simulink model "BallPlate_FLControl"  (R2018b)
settings: Solver=FixedStepAuto  StartTime=0.0  StopTime=20  FixedStep=0.01  RelTol=1e-5
undefined symbols (not defined in the file or in its folder): K
libraries: vrlib x42, simulink x5, aerolibanimutils x3, powerlib_meascontrol x1
(part 1 of 2)
settings Model: Creator=enrico  LastModifiedBy=Dan

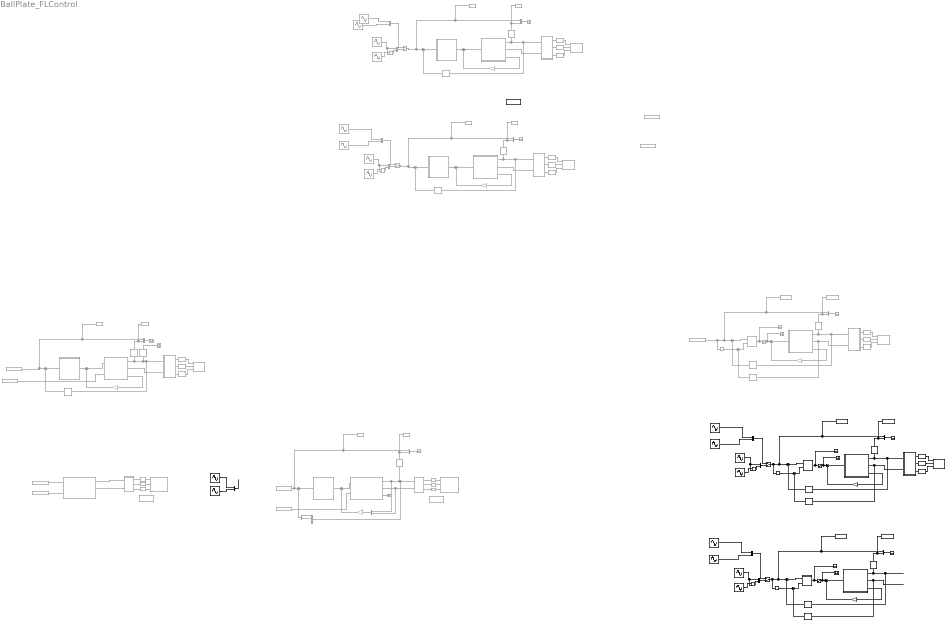
== system BallPlate_FLControl ==
  note: Controllo del sistema progettato sul linearizzato
  note: Visualization
  note: Visualization
  note: Visualization V1
  note: Visualization V1
  note: Visualization V1
  note: Visualization V1
  note: Visualization V1
  Constant1 : Constant  Commented=on  Value=[0.0001;0.0001;0.0;0.0]
  Constant2 : Constant  Commented=on  Value=[0.0001;0.0001;.0001;.0001]
  Constant3 : Constant  Commented=on  Value=[0;0.000000005]
  Constant4 : Constant  Commented=on  Value=[.24;-.24]
  Constant5 : Constant  Commented=on  Value=[0.24;0.2]
  Constant6 : Constant  Commented=on  Value=[.24;-.24]
  Constant7 : Constant  Commented=on  Value=[0.18;-0.24]
  Constant8 : Constant  Commented=on  Value=[.18; .24; 0.0001; 0.0001]
  Constant9 : Constant  Commented=on  Value=[0.18;-0.24]
  Control : Subsystem  Commented=on
  Control1 : Subsystem  Commented=on
  Control2 : Subsystem  Commented=on
  Control3 : Subsystem  Commented=on
  Demux1 : Demux  Commented=on
  Derivative : Derivative  Commented=on
  Derivative1 : Derivative
  Derivative2 : Derivative
  "Feedback linearized " : Subsystem  Commented=on
  Feedback linearized 1 : Subsystem  Commented=on
  Feedback linearized 2 : Subsystem  Commented=on
  Feedback linearized 3 : Subsystem  Commented=on
  Feedback linearized 4 : Subsystem
  Feedback linearized 5 : Subsystem
  Gain : Gain  Commented=on  Gain=K  Multiplication=Matrix(K*u)
  Gain{1..4} (4 alike) : Gain  Commented=on  Gain="[24,  50,   35,   10, 0, 0, 0, 0;  0, 0, 0, 0, 24,  50,  35, 10]"  Multiplication=Matrix(K*u)
  Gain5 : Gain  Gain="[24,  50,   35,   10, 0, 0, 0, 0;  0, 0, 0, 0, 24,  50,  35, 10]"  Multiplication=Matrix(K*u)
  Gain6 : Gain  Gain="[24,  50,   35,   10, 0, 0, 0, 0;  0, 0, 0, 0, 24,  50,  35, 10]"  Multiplication=Matrix(K*u)
  Manual Switch : ManualSwitch  Commented=on
  Manual Switch1 : ManualSwitch  Commented=on  CurrentSetting=0
  Manual Switch3 : ManualSwitch
  Manual Switch4 : ManualSwitch  CurrentSetting=0
  Mux{,1..2,4..11} (11 alike) : Mux  Commented=on  Inputs=2
  Mux{3,14..19} (7 alike) : Mux  Inputs=2
  Product : Product  Commented=on
  Product1 : Product  Commented=on
  Product3 : Product
  Product4 : Product
  Saturation : Saturate  Commented=on  UpperLimit=20  LowerLimit=-20
  Saturation1 : Saturate  UpperLimit=20  LowerLimit=-20
  Saturation2 : Saturate  UpperLimit=20  LowerLimit=-20
  Scope{,1..7} (8 alike) : Scope  Commented=on
  Scope{8..13} (6 alike) : Scope
  Selector{,1..6,8..10} (10 alike) : Selector  Commented=on  InputPortWidth=4  IndexOptions=Index vector (dialog)  Indices=[1 2]  OutputSizes=1
  Selector{11..16} (6 alike) : Selector  InputPortWidth=4  IndexOptions=Index vector (dialog)  Indices=[1 2]  OutputSizes=1
  Selector7 : Selector  Commented=on  InputPortWidth=4  IndexOptions=Index vector (dialog)  Indices=[3 4]  OutputSizes=1
  Simulation Pace1 : aerolibanimutils/Simulation Pace  Commented=on  SimulationPace=1  SleepMode=Auto  OutputPaceError=off  SampleTime=1/30
  Simulation Pace2 : aerolibanimutils/Simulation Pace  Commented=on  SimulationPace=1  SleepMode=Auto  OutputPaceError=off  SampleTime=1/30
  Simulation Pace3 : aerolibanimutils/Simulation Pace  SimulationPace=1  SleepMode=Auto  OutputPaceError=off  SampleTime=-1
  Sine Wave : Sin  Amplitude=.1  Frequency=.7  SampleTime=0
  Sine Wave1 : Sin  Amplitude=.1  Frequency=.7  Phase=pi/2  SampleTime=0
  Sine Wave14 : Sin  Amplitude=.26  SampleTime=0
  Sine Wave15 : Sin  Amplitude=1.2  Phase=pi/2  SampleTime=0
  Sine Wave16 : Sin  Amplitude=.23  SampleTime=0
  Sine Wave17 : Sin  Amplitude=0.23  Phase=pi/2  SampleTime=0
  Sine Wave18 : Sin  Amplitude=.26  SampleTime=0
  Sine Wave19 : Sin  Amplitude=1.2  Phase=pi/2  SampleTime=0
  Sine Wave{2,4,6,8} (4 alike) : Sin  Commented=on  Amplitude=.28  SampleTime=0
  Sine Wave20 : Sin  Amplitude=.23  SampleTime=0
  Sine Wave21 : Sin  Amplitude=0.23  Phase=pi/2  SampleTime=0
  Sine Wave3 : Sin  Commented=on  Amplitude=1.2  Phase=pi/2  SampleTime=0
  Sine Wave5 : Sin  Commented=on  Amplitude=0.28  Phase=pi/2  SampleTime=0
  Sine Wave7 : Sin  Commented=on  Amplitude=1.2  Phase=pi/2  SampleTime=0
  Sine Wave9 : Sin  Commented=on  Amplitude=0.28  Phase=pi/2  SampleTime=0
  Subsystem : Subsystem  Commented=on
  Subsystem1 : Subsystem  Commented=on
  Subsystem2 : Subsystem  Commented=on
  Subsystem3 : Subsystem
  Subsystem4 : Subsystem
  Sum{,1..10} (11 alike) : Sum  Commented=on  Inputs=|+-
  Sum{11..16} (6 alike) : Sum  Inputs=|+-
  Terminator1 : Terminator  Commented=on
  To Workspace : ToWorkspace  Commented=on  VariableName=xyref_circle  SampleTime=-1
  To Workspace1 : ToWorkspace  Commented=on  VariableName=xy_circle  SampleTime=-1
  To Workspace10 : ToWorkspace  VariableName=xyref_circular  SampleTime=-1
  To Workspace11 : ToWorkspace  VariableName=xy_circular  SampleTime=-1
  To Workspace12 : ToWorkspace  VariableName=xyref_infinity  SampleTime=-1
  To Workspace13 : ToWorkspace  VariableName=xy_infinity  SampleTime=-1
  To Workspace2 : ToWorkspace  Commented=on  VariableName=xyref_inf  SampleTime=-1
  To Workspace3 : ToWorkspace  Commented=on  VariableName=xy_inf  SampleTime=-1
  To Workspace4 : ToWorkspace  Commented=on  VariableName=xyref_PtoP  SampleTime=-1
  To Workspace5 : ToWorkspace  Commented=on  VariableName=xy_PtoP  SampleTime=-1
  To Workspace6 : ToWorkspace  Commented=on  VariableName=xyref_circle1  SampleTime=-1
  To Workspace7 : ToWorkspace  Commented=on  VariableName=xy_circle1  SampleTime=-1
  To Workspace8 : ToWorkspace  Commented=on  VariableName=xyref_PDG  SampleTime=-1
  To Workspace9 : ToWorkspace  Commented=on  VariableName=xy_PDG  SampleTime=-1
  VR Signal Expander{1,4,7,10,13,16} (6 alike) : vrlib/VR Signal Expander  Commented=on  outwidth=3  outidx=[1 2 3]
      settings: SourceProductName=Simulink 3D Animation  SourceProductBaseCode=VR
  VR Signal Expander{2..3,5..6,8..9,11..12,14..15,17..18} (12 alike) : vrlib/VR Signal Expander  Commented=on  outwidth=4  outidx=[1 2 3 4]
      settings: SourceProductName=Simulink 3D Animation  SourceProductBaseCode=VR
  VR Signal Expander19 : vrlib/VR Signal Expander  outwidth=3  outidx=[1 2 3]
      settings: SourceProductName=Simulink 3D Animation  SourceProductBaseCode=VR
  VR Signal Expander20 : vrlib/VR Signal Expander  outwidth=4  outidx=[1 2 3 4]
      settings: SourceProductName=Simulink 3D Animation  SourceProductBaseCode=VR
  VR Signal Expander21 : vrlib/VR Signal Expander  outwidth=4  outidx=[1 2 3 4]
      settings: SourceProductName=Simulink 3D Animation  SourceProductBaseCode=VR
  VR Sink{1..3,5} (4 alike) : vrlib/VR Sink  Commented=on  InstantiateOnLoad=on  SampleTime=-1  ViewEnable=on  RemoteChange=off  RemoteView=off  FieldsWritten=Ball.rotation.4.1.1.double#Ball.translation.3.1.1.double#Plate.rotation.4.1.1.double  WorldFileName=BallPlateVR.wrl  WorldDescription=Ball and plate  AutoView=on  VideoDimensions=[]  AllowVariableSize=off  mask(Virtual Reality Sink){}
      settings: SourceProductBaseCode=VR
  VR Sink4 : vrlib/VR Sink  Commented=on  InstantiateOnLoad=on  SampleTime=-1  ViewEnable=on  RemoteChange=off  RemoteView=off  FieldsWritten=Ball.rotation.4.1.1.double#Ball.translation.3.1.1.double#Plate.rotation.4.1.1.double  WorldFileName=BallPlateVR.wrl  WorldDescription=Ball and plate  AutoView=on  VideoDimensions=[]  AllowVariableSize=off  FigureProperties="{'Position', 'Name', 'Viewpoint', 'CameraBound', 'CameraDirection', 'CameraPosition', 'CameraUpVector', 'ZoomFactor', 'Antialiasing', 'Headlight', 'Lighting', 'NavPanel', 'Sound', 'StatusBar', 'Stereo3D', 'Stereo3DCameraOffset', 'Stereo3DHIT', 'ToolBar', 'Textures', 'Transparency', 'Triad', 'Wireframe', 'NavZones', 'NavMode', 'NavSpeed', 'CaptureFileFormat', 'CaptureFileName', 'Record2DCompressMethod', 'Record2DCompressQuality', 'Record2D', 'Record2DFileName', 'Record2DFPS'; [1.0000000000000000e+00   7.4199999999999932e+01   1.5360000000000000e+03   6.9880000000000007e+02], 'Ball and plate', '', 'on', [-1.8584785177561611e-02   9.6824130369892936e-01  -2.4932585820830763e-01], [1.8584785177561511e-01  -9.6824130369892938e+00   2.4932585820830795e+00], [-5.6033071681409391e-02   2.4796837288236298e-01   9.6714630792244927e-01], [2.5547669861876649e+01], 'on', 'on', 'on', 'halfbar', 'on', 'on', 'off', [1.0000000149011612e-01], [0.0000000000000000e+00], 'on', 'on', 'on', 'none', 'off', 'off', 'examine', 'normal', 'png', 'C:\\Users\\Dan\\Desktop\\DeltaRobot\\rep_delta\\TavoleControlloRobot\\Img\\BallAndBeamImg\\startframe.png', 'auto', [7.5000000000000000e+01], 'off', '%f_anim_%n.avi', 'auto'}"  mask(Virtual Reality Sink){}
      settings: SourceProductBaseCode=VR
  VR Sink6 : vrlib/VR Sink  Commented=on  InstantiateOnLoad=on  SampleTime=-1  ViewEnable=on  RemoteChange=off  RemoteView=off  FieldsWritten=Ball.rotation.4.1.1.double#Ball.translation.3.1.1.double#Plate.rotation.4.1.1.double  WorldFileName=BallPlateVR.wrl  WorldDescription=Ball and plate  AutoView=on  VideoDimensions=[]  AllowVariableSize=off  FigureProperties="{'Position', 'Name', 'Viewpoint', 'CameraBound', 'CameraDirection', 'CameraPosition', 'CameraUpVector', 'ZoomFactor', 'Antialiasing', 'Headlight', 'Lighting', 'NavPanel', 'Sound', 'StatusBar', 'Stereo3D', 'Stereo3DCameraOffset', 'Stereo3DHIT', 'ToolBar', 'Textures', 'Transparency', 'Triad', 'Wireframe', 'NavZones', 'NavMode', 'NavSpeed', 'CaptureFileFormat', 'CaptureFileName', 'Record2DCompressMethod', 'Record2DCompressQuality', 'Record2D', 'Record2DFileName', 'Record2DFPS'; [5.0000000000000000e+00   9.2000000000000000e+01   5.7600000000000000e+02   3.5000000000000000e+02], 'Ball and plate', '', 'on', [-9.4945185305419899e-02   9.6436406829919863e-01  -2.4695618145886314e-01], [9.4945185305419966e-01  -9.6436406829919896e+00   2.4695618145886380e+00], [2.4301361782686895e-02   2.5024825439514964e-01   9.6787667343917927e-01], [1.5863092971714948e+01], 'on', 'on', 'on', 'halfbar', 'on', 'on', 'off', [1.0000000149011612e-01], [0.0000000000000000e+00], 'on', 'on', 'on', 'none', 'off', 'off', 'examine', 'normal', 'tif', '%f_anim_%n.tif', 'auto', [7.5000000000000000e+01], 'off', '%f_anim_%n.avi', 'auto'}"  mask(Virtual Reality Sink){}
      settings: SourceProductBaseCode=VR
  VR Sink7 : vrlib/VR Sink  InstantiateOnLoad=on  SampleTime=-1  ViewEnable=on  RemoteChange=off  RemoteView=off  FieldsWritten=Ball.rotation.4.1.1.double#Ball.translation.3.1.1.double#Plate.rotation.4.1.1.double  WorldFileName=BallPlateVR.wrl  WorldDescription=Ball and plate  AutoView=on  VideoDimensions=[]  AllowVariableSize=off  mask(Virtual Reality Sink){}
      settings: SourceProductBaseCode=VR
  Visualization parsing1 : Subsystem  Commented=on
  Visualization parsing2 : Subsystem  Commented=on
  Visualization parsing3 : Subsystem  Commented=on
  Visualization parsing4 : Subsystem  Commented=on
  Visualization parsing5 : Subsystem  Commented=on
  Visualization parsing6 : Subsystem  Commented=on
  Visualization parsing7 : Subsystem
  wires:
  Control/1(nu) -> Sum3/1
  Sum/1 -> Control/1(e)
  Gain/1 -> Sum2/2
  Demux1/1 -> Mux1/1
  Demux1/2 -> Mux1/2
  Control1/1(nu) -> Sum2/1
  Subsystem1/3(ddq) -> Terminator1/1
  Mux1/1 -> Sum1/2  "x,y"
  Sum1/1 -> Control1/1(e)
  Mux2/1 -> Gain/1  "x,y"
  Sum2/1 -> Subsystem1/1(tau)
  Sine Wave/1 -> Mux3/1
  Sine Wave1/1 -> Mux3/2
  Mux3/1 -> ?  "x,y"
  Sum3/1 -> "Feedback linearized "/1(nu)
  "Feedback linearized "/3(z) -> Gain1/1
  Gain1/1 -> Sum3/2
  Sine Wave2/1 -> Product/2, Mux4/1
  Sine Wave3/1 -> Product/1
  Manual Switch/1 -> To Workspace/1, Mux/1, Sum/1  "x,y"
  Subsystem1/2(dq) -> Visualization parsing1/2(dq), Mux2/2
  Visualization parsing1/3(Plate rot) -> VR Signal Expander5/1
  Visualization parsing1/2(xyz) -> VR Signal Expander4/1
  Subsystem1/1(q) -> Mux2/1, Selector6/1, Visualization parsing1/1(q), Demux1/1
  Visualization parsing1/1(Ball rot) -> VR Signal Expander3/1
  VR Signal Expander5/1 -> VR Sink1/3
  VR Signal Expander3/1 -> VR Sink1/1
  VR Signal Expander4/1 -> VR Sink1/2
  Subsystem2/2(dq) -> Visualization parsing2/2(dq)
  Visualization parsing2/3(Plate rot) -> VR Signal Expander8/1
  Visualization parsing2/2(xyz) -> VR Signal Expander7/1
  Subsystem2/1(q) -> Visualization parsing2/1(q)
  Visualization parsing2/1(Ball rot) -> VR Signal Expander6/1
  VR Signal Expander8/1 -> VR Sink2/3
  VR Signal Expander6/1 -> VR Sink2/1
  VR Signal Expander7/1 -> VR Sink2/2
  Constant1/1 -> Subsystem2/2(Input)
  Constant3/1 -> Subsystem2/1(tau)
  Visualization parsing3/3(Plate rot) -> VR Signal Expander11/1
  "Feedback linearized "/1(q) -> Selector1/1, Selector/1, Visualization parsing3/1(q)
  VR Signal Expander9/1 -> VR Sink3/1
  Visualization parsing3/2(xyz) -> VR Signal Expander10/1
  Visualization parsing3/1(Ball rot) -> VR Signal Expander9/1
  "Feedback linearized "/2(dq) -> Visualization parsing3/2(dq)
  VR Signal Expander10/1 -> VR Sink3/2
  VR Signal Expander11/1 -> VR Sink3/3
  Product/1 -> Mux4/2
  Selector/1 -> Sum/2
  Mux/1 -> Scope/1
  Constant2/1 -> Subsystem1/2(Input)
  Mux4/1 -> Manual Switch/2  "x,y"
  Mux5/1 -> Manual Switch/1
  Sine Wave4/1 -> Mux5/2
  Sine Wave5/1 -> Mux5/1
  Sine Wave9/1 -> Mux8/1
  Sine Wave8/1 -> Mux8/2
  Mux8/1 -> Manual Switch1/1
  Mux7/1 -> Manual Switch1/2  "x,y"
  Mux6/1 -> Scope1/1
  Selector2/1 -> Sum4/2
  Product1/1 -> Mux7/2
  VR Signal Expander2/1 -> VR Sink4/3
  VR Signal Expander1/1 -> VR Sink4/2
  Feedback linearized 1/2(dq) -> Visualization parsing4/2(dq)
  Visualization parsing4/1(Ball rot) -> VR Signal Expander12/1
  Visualization parsing4/2(xyz) -> VR Signal Expander1/1
  VR Signal Expander12/1 -> VR Sink4/1
  Feedback linearized 1/1(q) -> Visualization parsing4/1(q), Selector2/1, Selector3/1
  Visualization parsing4/3(Plate rot) -> VR Signal Expander2/1
  Sine Wave7/1 -> Product1/1
  Sine Wave6/1 -> Mux7/1, Product1/2
  Gain2/1 -> Sum5/2
  Feedback linearized 1/3(z) -> Gain2/1
  Sum5/1 -> Feedback linearized 1/1(nu)
  Sum4/1 -> Control2/1(e)
  Control2/1(nu) -> Sum5/1
  Selector1/1 -> Mux/2, To Workspace1/1
  Selector3/1 -> To Workspace3/1, Mux6/2
  Manual Switch1/1 -> Sum4/1, To Workspace2/1, Mux6/1  "x,y"
  Constant7/1 -> Mux9/1, To Workspace4/1, Sum6/1  "x,y"
  Selector5/1 -> Mux9/2, To Workspace5/1
  Control3/1(nu) -> Sum7/1
  Sum6/1 -> Control3/1(e)
  Sum7/1 -> Feedback linearized 2/1(nu)
  Feedback linearized 2/3(z) -> Gain3/1
  Gain3/1 -> Sum7/2
  Visualization parsing5/3(Plate rot) -> VR Signal Expander15/1
  Feedback linearized 2/1(q) -> Selector5/1, Selector7/1, Selector4/1, Visualization parsing5/1(q)
  VR Signal Expander14/1 -> VR Sink5/1
  Visualization parsing5/2(xyz) -> VR Signal Expander13/1
  Visualization parsing5/1(Ball rot) -> VR Signal Expander14/1
  Feedback linearized 2/2(dq) -> Visualization parsing5/2(dq)
  VR Signal Expander13/1 -> VR Sink5/2
  VR Signal Expander15/1 -> VR Sink5/3
  Selector4/1 -> Sum6/2
  Mux9/1 -> Scope2/1
  Constant8/1 -> Feedback linearized 2/2("p0 ")  "x,y"
  Selector6/1 -> Mux10/2, To Workspace7/1
  Constant5/1 -> Mux10/1, To Workspace6/1, Sum1/1  "x,y"
  Mux10/1 -> Scope3/1
  Selector7/1 -> Scope4/1
  Constant9/1 -> Derivative/1, Mux11/1, To Workspace8/1, Sum8/1  "x,y"
  Selector9/1 -> Mux11/2, To Workspace9/1
  Sum8/1 -> Subsystem/1(In1)
  Sum9/1 -> Feedback linearized 3/1(nu)
  Feedback linearized 3/3(z) -> Gain4/1
  Gain4/1 -> Sum9/2
  Visualization parsing6/3(Plate rot) -> VR Signal Expander18/1
  Feedback linearized 3/1(q) -> Selector9/1, Selector8/1, Visualization parsing6/1(q)
  VR Signal Expander17/1 -> VR Sink6/1
  Visualization parsing6/2(xyz) -> VR Signal Expander16/1
  Visualization parsing6/1(Ball rot) -> VR Signal Expander17/1
  Feedback linearized 3/2(dq) -> Selector10/1, Visualization parsing6/2(dq)
  VR Signal Expander16/1 -> VR Sink6/2
  VR Signal Expander18/1 -> VR Sink6/3
  Selector8/1 -> Sum8/2
  Mux11/1 -> Scope5/1
  Selector10/1 -> Sum10/2
  Subsystem/1(Out1) -> Saturation/1, Scope6/1
  Derivative/1 -> Sum10/1
  Sum10/1 -> Subsystem/2(In2)
  Saturation/1 -> Scope7/1, Sum9/1
  Saturation1/1 -> Sum13/1, Scope10/1
  Sum11/1 -> Subsystem3/2(In2)
  Derivative1/1 -> Sum11/1
  Subsystem3/1(Out1) -> Scope9/1, Saturation1/1
  Selector11/1 -> Sum11/2
  Sine Wave17/1 -> Mux16/1
  Sine Wave16/1 -> Mux16/2
  Mux16/1 -> Manual Switch3/1
  Mux15/1 -> Manual Switch3/2  "x,y"
  Mux14/1 -> Scope8/1
  Selector12/1 -> Sum12/2
  Product3/1 -> Mux15/2
  Feedback linearized 4/2(dq) -> Visualization parsing7/2(dq), Selector11/1
  Feedback linearized 4/1(q) -> Visualization parsing7/1(q), Selector12/1, Selector13/1
  Sine Wave15/1 -> Product3/1
  Sine Wave14/1 -> Mux15/1, Product3/2
  Gain5/1 -> Sum13/2
  Feedback linearized 4/3(z) -> Gain5/1
  Sum13/1 -> Feedback linearized 4/1(nu)
  Sum12/1 -> Subsystem3/1(In1)
  Selector13/1 -> To Workspace11/1, Mux14/2
  Manual Switch3/1 -> Sum12/1, To Workspace10/1, Mux14/1, Derivative1/1  "x,y"
  Manual Switch4/1 -> Derivative2/1, Mux17/1, To Workspace12/1, Sum15/1  "x,y"
  Selector16/1 -> Mux17/2, To Workspace13/1
  Sum15/1 -> Subsystem4/1(In1)
  Sum16/1 -> Feedback linearized 5/1(nu)
  Feedback linearized 5/3(z) -> Gain6/1
  Gain6/1 -> Sum16/2
  Sine Wave18/1 -> Product4/2, Mux18/1
  Sine Wave19/1 -> Product4/1
  Feedback linearized 5/1(q) -> Selector16/1, Selector15/1
  Feedback linearized 5/2(dq) -> Selector14/1
  Product4/1 -> Mux18/2
  Selector15/1 -> Sum15/2
  Mux17/1 -> Scope12/1
  Mux18/1 -> Manual Switch4/2  "x,y"
  Mux19/1 -> Manual Switch4/1
  Sine Wave20/1 -> Mux19/2
  Sine Wave21/1 -> Mux19/1
  Selector14/1 -> Sum14/2
  Subsystem4/1(Out1) -> Saturation2/1, Scope13/1
  Derivative2/1 -> Sum14/1
  Sum14/1 -> Subsystem4/2(In2)
  Saturation2/1 -> Scope11/1, Sum16/1
  VR Signal Expander21/1 -> VR Sink7/3
  VR Signal Expander19/1 -> VR Sink7/2
  Visualization parsing7/1(Ball rot) -> VR Signal Expander20/1
  Visualization parsing7/2(xyz) -> VR Signal Expander19/1
  VR Signal Expander20/1 -> VR Sink7/1
  Visualization parsing7/3(Plate rot) -> VR Signal Expander21/1

== system BallPlate_FLControl/Control ==
  e : Inport
  Demux : Demux  Outputs=2
  Mux : Mux  Inputs=2
  PID Controller1 : simulink/Continuous/PID Controller  Controller=PID  Form=Parallel  TimeDomain=Continuous-time  SampleTime=-1  IntegratorMethod=Forward Euler  FilterMethod=Forward Euler  ControllerParametersSource=internal  P=82.8802  I=28.8647  D=59.4942  UseFilter=on  N=100  TunerSelectOption=Transfer Function Based (PID Tuner App)  InitialConditionSource=internal  InitialConditionForIntegrator=0  InitialConditionForFilter=0  DifferentiatorICPrevScaledInput=0  ExternalReset=none  TrackingMode=off  Kt=1  LimitOutput=off  UpperSaturationLimit=inf  LowerSaturationLimit=-inf  LinearizeAsGain=on  AntiWindupMode=none  Kb=1  POutMin=[]  POutMax=[]  IOutMin=[]  IOutMax=[]  DOutMin=[]  DOutMax=[]  NOutMin=[]  NOutMax=[]  SumOutMin=[]  SumOutMax=[]  SaturationOutMin=[]  SaturationOutMax=[]  PParamMin=[]  PParamMax=[]  IParamMin=[]  IParamMax=[]  DParamMin=[]  DParamMax=[]  NParamMin=[]  NParamMax=[]  KbParamMin=[]  KbParamMax=[]  KtParamMin=[]  KtParamMax=[]  KbOutMin=[]  KbOutMax=[]  KtOutMin=[]  KtOutMax=[]  IntegratorOutMin=[]  IntegratorOutMax=[]  FilterOutMin=[]  FilterOutMax=[]  SumI1OutMin=[]  SumI1OutMax=[]  SumI2OutMin=[]  SumI2OutMax=[]  SumI3OutMin=[]  SumI3OutMax=[]  SumI4OutMin=[]  SumI4OutMax=[]  SumDOutMin=[]  SumDOutMax=[]  DifferentiatorOutMin=[]  DifferentiatorOutMax=[]  FilterDiffOutCoefMin=[]  FilterDiffOutCoefMax=[]  ReciprocalOutMin=[]  ReciprocalOutMax=[]  SumDenOutMin=[]  SumDenOutMax=[]  SumNumOutMin=[]  SumNumOutMax=[]  DivideOutMin=[]  DivideOutMax=[]  IntegratorContinuousStateAttributes=''  IntegratorStateMustResolveToSignalObject=off  IntegratorRTWStateStorageClass=Auto  FilterContinuousStateAttributes=''  FilterStateMustResolveToSignalObject=off  FilterRTWStateStorageClass=Auto  ParallelPVariant=InternalParameters  IdealPVariant=Disabled  IVariant=InternalParameters  DVariant=InternalParameters  IntegratorVariant=Continuous  SatVariant=Disabled  AWVariant=Passthrough  PCopyVariant=Disabled  TRVariant=Disabled  FdbkBlocksVariant=Forward  IdealPFdbkVariant=Disabled  SatFdbkVariant=Disabled  DerivativeFilterVariant=ContFilter  NVariant=InternalParameters  NCopyVariant=Disabled  FilterICVariant=InternalICsFilter  IntegratorICVariant=InternalICs  ExternalResetVariant=Disabled  TRSumVariant=Passthrough  SumFdbkVariant=Disabled  SumVariant=Sum_PID
  PID Controller2 : simulink/Continuous/PID Controller  Commented=on  Controller=PID  Form=Parallel  TimeDomain=Continuous-time  SampleTime=-1  IntegratorMethod=Forward Euler  FilterMethod=Forward Euler  ControllerParametersSource=internal  P=80.2018  I=30.9918  D=0.1897  UseFilter=on  N=0.0039901  TunerSelectOption=Transfer Function Based (PID Tuner App)  InitialConditionSource=internal  InitialConditionForIntegrator=0  InitialConditionForFilter=0  DifferentiatorICPrevScaledInput=0  ExternalReset=none  TrackingMode=off  Kt=1  LimitOutput=off  UpperSaturationLimit=inf  LowerSaturationLimit=-inf  LinearizeAsGain=on  AntiWindupMode=none  Kb=1  POutMin=[]  POutMax=[]  IOutMin=[]  IOutMax=[]  DOutMin=[]  DOutMax=[]  NOutMin=[]  NOutMax=[]  SumOutMin=[]  SumOutMax=[]  SaturationOutMin=[]  SaturationOutMax=[]  PParamMin=[]  PParamMax=[]  IParamMin=[]  IParamMax=[]  DParamMin=[]  DParamMax=[]  NParamMin=[]  NParamMax=[]  KbParamMin=[]  KbParamMax=[]  KtParamMin=[]  KtParamMax=[]  KbOutMin=[]  KbOutMax=[]  KtOutMin=[]  KtOutMax=[]  IntegratorOutMin=[]  IntegratorOutMax=[]  FilterOutMin=[]  FilterOutMax=[]  SumI1OutMin=[]  SumI1OutMax=[]  SumI2OutMin=[]  SumI2OutMax=[]  SumI3OutMin=[]  SumI3OutMax=[]  SumI4OutMin=[]  SumI4OutMax=[]  SumDOutMin=[]  SumDOutMax=[]  DifferentiatorOutMin=[]  DifferentiatorOutMax=[]  FilterDiffOutCoefMin=[]  FilterDiffOutCoefMax=[]  ReciprocalOutMin=[]  ReciprocalOutMax=[]  SumDenOutMin=[]  SumDenOutMax=[]  SumNumOutMin=[]  SumNumOutMax=[]  DivideOutMin=[]  DivideOutMax=[]  IntegratorContinuousStateAttributes=''  IntegratorStateMustResolveToSignalObject=off  IntegratorRTWStateStorageClass=Auto  FilterContinuousStateAttributes=''  FilterStateMustResolveToSignalObject=off  FilterRTWStateStorageClass=Auto  ParallelPVariant=InternalParameters  IdealPVariant=Disabled  IVariant=InternalParameters  DVariant=InternalParameters  IntegratorVariant=Continuous  SatVariant=Disabled  AWVariant=Passthrough  PCopyVariant=Disabled  TRVariant=Disabled  FdbkBlocksVariant=Forward  IdealPFdbkVariant=Disabled  SatFdbkVariant=Disabled  DerivativeFilterVariant=ContFilter  NVariant=InternalParameters  NCopyVariant=Disabled  FilterICVariant=InternalICsFilter  IntegratorICVariant=InternalICs  ExternalResetVariant=Disabled  TRSumVariant=Passthrough  SumFdbkVariant=Disabled  SumVariant=Sum_PID
  PID Controller4 : simulink/Continuous/PID Controller  Controller=PID  Form=Parallel  TimeDomain=Continuous-time  SampleTime=-1  IntegratorMethod=Forward Euler  FilterMethod=Forward Euler  ControllerParametersSource=internal  P=82.8802  I=28.8647  D=59.4942  UseFilter=on  N=100  TunerSelectOption=Transfer Function Based (PID Tuner App)  InitialConditionSource=internal  InitialConditionForIntegrator=0  InitialConditionForFilter=0  DifferentiatorICPrevScaledInput=0  ExternalReset=none  TrackingMode=off  Kt=1  LimitOutput=off  UpperSaturationLimit=inf  LowerSaturationLimit=-inf  LinearizeAsGain=on  AntiWindupMode=none  Kb=1  POutMin=[]  POutMax=[]  IOutMin=[]  IOutMax=[]  DOutMin=[]  DOutMax=[]  NOutMin=[]  NOutMax=[]  SumOutMin=[]  SumOutMax=[]  SaturationOutMin=[]  SaturationOutMax=[]  PParamMin=[]  PParamMax=[]  IParamMin=[]  IParamMax=[]  DParamMin=[]  DParamMax=[]  NParamMin=[]  NParamMax=[]  KbParamMin=[]  KbParamMax=[]  KtParamMin=[]  KtParamMax=[]  KbOutMin=[]  KbOutMax=[]  KtOutMin=[]  KtOutMax=[]  IntegratorOutMin=[]  IntegratorOutMax=[]  FilterOutMin=[]  FilterOutMax=[]  SumI1OutMin=[]  SumI1OutMax=[]  SumI2OutMin=[]  SumI2OutMax=[]  SumI3OutMin=[]  SumI3OutMax=[]  SumI4OutMin=[]  SumI4OutMax=[]  SumDOutMin=[]  SumDOutMax=[]  DifferentiatorOutMin=[]  DifferentiatorOutMax=[]  FilterDiffOutCoefMin=[]  FilterDiffOutCoefMax=[]  ReciprocalOutMin=[]  ReciprocalOutMax=[]  SumDenOutMin=[]  SumDenOutMax=[]  SumNumOutMin=[]  SumNumOutMax=[]  DivideOutMin=[]  DivideOutMax=[]  IntegratorContinuousStateAttributes=''  IntegratorStateMustResolveToSignalObject=off  IntegratorRTWStateStorageClass=Auto  FilterContinuousStateAttributes=''  FilterStateMustResolveToSignalObject=off  FilterRTWStateStorageClass=Auto  ParallelPVariant=InternalParameters  IdealPVariant=Disabled  IVariant=InternalParameters  DVariant=InternalParameters  IntegratorVariant=Continuous  SatVariant=Disabled  AWVariant=Passthrough  PCopyVariant=Disabled  TRVariant=Disabled  FdbkBlocksVariant=Forward  IdealPFdbkVariant=Disabled  SatFdbkVariant=Disabled  DerivativeFilterVariant=ContFilter  NVariant=InternalParameters  NCopyVariant=Disabled  FilterICVariant=InternalICsFilter  IntegratorICVariant=InternalICs  ExternalResetVariant=Disabled  TRSumVariant=Passthrough  SumFdbkVariant=Disabled  SumVariant=Sum_PID
  nu : Outport
  wires:
  e/1 -> Demux/1
  PID Controller4/1 -> Mux/1
  Mux/1 -> nu/1
  Demux/1 -> PID Controller4/1
  Demux/2 -> PID Controller1/1
  PID Controller1/1 -> Mux/2

== system BallPlate_FLControl/Control1 ==
  e : Inport
  Gain : Gain  Gain=-3
  Integrator : Integrator
  nu : Outport
  wires:
  Gain/1 -> Integrator/1
  Integrator/1 -> nu/1
  e/1 -> Gain/1

== system BallPlate_FLControl/Control2 ==
  e : Inport
  Demux : Demux  Outputs=2
  Lead-Lag Filter : powerlib_meascontrol/Filters/Lead-Lag Filter  T1=5e-3  T2=20e-3  Vdc_Init=0  Ts=0
      settings: SourceProductName=Simscape Power Systems  SourceProductBaseCode=PS
  Mux : Mux  Inputs=2
  PID Controller1 : simulink/Continuous/PID Controller  Controller=PID  Form=Parallel  TimeDomain=Continuous-time  SampleTime=-1  IntegratorMethod=Forward Euler  FilterMethod=Forward Euler  ControllerParametersSource=internal  P=82.8802  I=28.8647  D=59.4942  UseFilter=on  N=100  TunerSelectOption=Transfer Function Based (PID Tuner App)  InitialConditionSource=internal  InitialConditionForIntegrator=0  InitialConditionForFilter=0  DifferentiatorICPrevScaledInput=0  ExternalReset=none  TrackingMode=off  Kt=1  LimitOutput=off  UpperSaturationLimit=inf  LowerSaturationLimit=-inf  LinearizeAsGain=on  AntiWindupMode=none  Kb=1  POutMin=[]  POutMax=[]  IOutMin=[]  IOutMax=[]  DOutMin=[]  DOutMax=[]  NOutMin=[]  NOutMax=[]  SumOutMin=[]  SumOutMax=[]  SaturationOutMin=[]  SaturationOutMax=[]  PParamMin=[]  PParamMax=[]  IParamMin=[]  IParamMax=[]  DParamMin=[]  DParamMax=[]  NParamMin=[]  NParamMax=[]  KbParamMin=[]  KbParamMax=[]  KtParamMin=[]  KtParamMax=[]  KbOutMin=[]  KbOutMax=[]  KtOutMin=[]  KtOutMax=[]  IntegratorOutMin=[]  IntegratorOutMax=[]  FilterOutMin=[]  FilterOutMax=[]  SumI1OutMin=[]  SumI1OutMax=[]  SumI2OutMin=[]  SumI2OutMax=[]  SumI3OutMin=[]  SumI3OutMax=[]  SumI4OutMin=[]  SumI4OutMax=[]  SumDOutMin=[]  SumDOutMax=[]  DifferentiatorOutMin=[]  DifferentiatorOutMax=[]  FilterDiffOutCoefMin=[]  FilterDiffOutCoefMax=[]  ReciprocalOutMin=[]  ReciprocalOutMax=[]  SumDenOutMin=[]  SumDenOutMax=[]  SumNumOutMin=[]  SumNumOutMax=[]  DivideOutMin=[]  DivideOutMax=[]  IntegratorContinuousStateAttributes=''  IntegratorStateMustResolveToSignalObject=off  IntegratorRTWStateStorageClass=Auto  FilterContinuousStateAttributes=''  FilterStateMustResolveToSignalObject=off  FilterRTWStateStorageClass=Auto  ParallelPVariant=InternalParameters  IdealPVariant=Disabled  IVariant=InternalParameters  DVariant=InternalParameters  IntegratorVariant=Continuous  SatVariant=Disabled  AWVariant=Passthrough  PCopyVariant=Disabled  TRVariant=Disabled  FdbkBlocksVariant=Forward  IdealPFdbkVariant=Disabled  SatFdbkVariant=Disabled  DerivativeFilterVariant=ContFilter  NVariant=InternalParameters  NCopyVariant=Disabled  FilterICVariant=InternalICsFilter  IntegratorICVariant=InternalICs  ExternalResetVariant=Disabled  TRSumVariant=Passthrough  SumFdbkVariant=Disabled  SumVariant=Sum_PID
  PID Controller2 : simulink/Continuous/PID Controller  Controller=PID  Form=Parallel  TimeDomain=Continuous-time  SampleTime=-1  IntegratorMethod=Forward Euler  FilterMethod=Forward Euler  ControllerParametersSource=internal  P=82.8802  I=28.8647  D=59.4942  UseFilter=on  N=100  TunerSelectOption=Transfer Function Based (PID Tuner App)  InitialConditionSource=internal  InitialConditionForIntegrator=0  InitialConditionForFilter=0  DifferentiatorICPrevScaledInput=0  ExternalReset=none  TrackingMode=off  Kt=1  LimitOutput=off  UpperSaturationLimit=inf  LowerSaturationLimit=-inf  LinearizeAsGain=on  AntiWindupMode=none  Kb=1  POutMin=[]  POutMax=[]  IOutMin=[]  IOutMax=[]  DOutMin=[]  DOutMax=[]  NOutMin=[]  NOutMax=[]  SumOutMin=[]  SumOutMax=[]  SaturationOutMin=[]  SaturationOutMax=[]  PParamMin=[]  PParamMax=[]  IParamMin=[]  IParamMax=[]  DParamMin=[]  DParamMax=[]  NParamMin=[]  NParamMax=[]  KbParamMin=[]  KbParamMax=[]  KtParamMin=[]  KtParamMax=[]  KbOutMin=[]  KbOutMax=[]  KtOutMin=[]  KtOutMax=[]  IntegratorOutMin=[]  IntegratorOutMax=[]  FilterOutMin=[]  FilterOutMax=[]  SumI1OutMin=[]  SumI1OutMax=[]  SumI2OutMin=[]  SumI2OutMax=[]  SumI3OutMin=[]  SumI3OutMax=[]  SumI4OutMin=[]  SumI4OutMax=[]  SumDOutMin=[]  SumDOutMax=[]  DifferentiatorOutMin=[]  DifferentiatorOutMax=[]  FilterDiffOutCoefMin=[]  FilterDiffOutCoefMax=[]  ReciprocalOutMin=[]  ReciprocalOutMax=[]  SumDenOutMin=[]  SumDenOutMax=[]  SumNumOutMin=[]  SumNumOutMax=[]  DivideOutMin=[]  DivideOutMax=[]  IntegratorContinuousStateAttributes=''  IntegratorStateMustResolveToSignalObject=off  IntegratorRTWStateStorageClass=Auto  FilterContinuousStateAttributes=''  FilterStateMustResolveToSignalObject=off  FilterRTWStateStorageClass=Auto  ParallelPVariant=InternalParameters  IdealPVariant=Disabled  IVariant=InternalParameters  DVariant=InternalParameters  IntegratorVariant=Continuous  SatVariant=Disabled  AWVariant=Passthrough  PCopyVariant=Disabled  TRVariant=Disabled  FdbkBlocksVariant=Forward  IdealPFdbkVariant=Disabled  SatFdbkVariant=Disabled  DerivativeFilterVariant=ContFilter  NVariant=InternalParameters  NCopyVariant=Disabled  FilterICVariant=InternalICsFilter  IntegratorICVariant=InternalICs  ExternalResetVariant=Disabled  TRSumVariant=Passthrough  SumFdbkVariant=Disabled  SumVariant=Sum_PID
  nu : Outport
  wires:
  PID Controller1/1 -> Mux/2
  PID Controller2/1 -> Mux/1
  Demux/2 -> PID Controller1/1
  Demux/1 -> PID Controller2/1
  Mux/1 -> nu/1
  e/1 -> Lead-Lag Filter/1
  Lead-Lag Filter/1 -> Demux/1

== system BallPlate_FLControl/Control3 ==
  e : Inport
  Demux : Demux  Outputs=2
  Gain : Gain  Gain=50
  Integrator : Integrator
  Integrator1 : Integrator
  Mux : Mux  Inputs=2
  nu : Outport
  wires:
  e/1 -> Demux/1
  Demux/1 -> Integrator/1
  Demux/2 -> Integrator1/1
  Integrator/1 -> Mux/1
  Integrator1/1 -> Mux/2
  Mux/1 -> Gain/1
  Gain/1 -> nu/1

== system BallPlate_FLControl/Feedback linearized  ==
  nu : Inport
  Coordinate transform : MATLAB Function  TreatAsAtomicUnit=on
  Feedback Linearization : Subsystem
  Subsystem : Subsystem
  q : Outport
  dq : Outport  Port=2
  z : Outport  Port=3
  wires:
  Feedback Linearization/1(u) -> Subsystem/1(tau)
  Subsystem/2(dq) -> Coordinate transform/2(dq), dq/1, Feedback Linearization/3(dq)
  nu/1 -> Feedback Linearization/1(nu)
  Subsystem/1(q) -> Coordinate transform/1(q), q/1, Feedback Linearization/2(q)
  Coordinate transform/1(z) -> z/1

== system BallPlate_FLControl/Feedback linearized 1 ==
  nu : Inport
  Coordinate transform : MATLAB Function  TreatAsAtomicUnit=on
  Feedback Linearization : Subsystem
  Subsystem : Subsystem
  q : Outport
  dq : Outport  Port=2
  z : Outport  Port=3
  wires:
  Coordinate transform/1(z) -> z/1
  Subsystem/1(q) -> Feedback Linearization/2(q), q/1, Coordinate transform/1(q)
  nu/1 -> Feedback Linearization/1(nu)
  Subsystem/2(dq) -> Feedback Linearization/3(dq), dq/1, Coordinate transform/2(dq)
  Feedback Linearization/1(u) -> Subsystem/1(tau)

== system BallPlate_FLControl/Feedback linearized 2 ==
  nu : Inport
  "p0 " : Inport  Port=2
  Coordinate transform : MATLAB Function  TreatAsAtomicUnit=on
  Feedback Linearization : Subsystem
  Subsystem : Subsystem
  q : Outport
  dq : Outport  Port=2
  z : Outport  Port=3
  wires:
  Feedback Linearization/1(u) -> Subsystem/1(tau)
  Subsystem/2(dq) -> Coordinate transform/2(dq), dq/1, Feedback Linearization/3(dq)
  nu/1 -> Feedback Linearization/1(nu)
  Subsystem/1(q) -> Coordinate transform/1(q), q/1, Feedback Linearization/2(q)
  Coordinate transform/1(z) -> z/1
  "p0 "/1 -> Subsystem/2("p0 ")

== system BallPlate_FLControl/Feedback linearized 3 ==
  nu : Inport
  Coordinate transform : MATLAB Function  TreatAsAtomicUnit=on
  Feedback Linearization : Subsystem
  Subsystem : Subsystem
  q : Outport
  dq : Outport  Port=2
  z : Outport  Port=3
  wires:
  Feedback Linearization/1(u) -> Subsystem/1(tau)
  Subsystem/2(dq) -> Coordinate transform/2(dq), dq/1, Feedback Linearization/3(dq)
  nu/1 -> Feedback Linearization/1(nu)
  Subsystem/1(q) -> Coordinate transform/1(q), q/1, Feedback Linearization/2(q)
  Coordinate transform/1(z) -> z/1

== system BallPlate_FLControl/Feedback linearized 4 ==
  nu : Inport
  Coordinate transform : MATLAB Function  TreatAsAtomicUnit=on
  Feedback Linearization : Subsystem
  Subsystem : Subsystem
  q : Outport
  dq : Outport  Port=2
  z : Outport  Port=3
  wires:
  Coordinate transform/1(z) -> z/1
  Subsystem/1(q) -> Feedback Linearization/2(q), q/1, Coordinate transform/1(q)
  nu/1 -> Feedback Linearization/1(nu)
  Subsystem/2(dq) -> Feedback Linearization/3(dq), dq/1, Coordinate transform/2(dq)
  Feedback Linearization/1(u) -> Subsystem/1(tau)

== system BallPlate_FLControl/Feedback linearized 5 ==
  nu : Inport
  Coordinate transform : MATLAB Function  TreatAsAtomicUnit=on
  Feedback Linearization : Subsystem
  Subsystem : Subsystem
  q : Outport
  dq : Outport  Port=2
  z : Outport  Port=3
  wires:
  Feedback Linearization/1(u) -> Subsystem/1(tau)
  Subsystem/2(dq) -> Coordinate transform/2(dq), dq/1, Feedback Linearization/3(dq)
  nu/1 -> Feedback Linearization/1(nu)
  Subsystem/1(q) -> Coordinate transform/1(q), q/1, Feedback Linearization/2(q)
  Coordinate transform/1(z) -> z/1

== system BallPlate_FLControl/Subsystem ==
  In1 : Inport
  In2 : Inport  Port=2
  Gain : Gain  Gain=100
  Gain1 : Gain  Gain=2000
  Integrator : Integrator
  Sum : Sum  Inputs=|++
  Out1 : Outport
  wires:
  In1/1 -> Gain/1
  In2/1 -> Gain1/1
  Sum/1 -> Integrator/1
  Integrator/1 -> Out1/1
  Gain/1 -> Sum/1
  Gain1/1 -> Sum/2

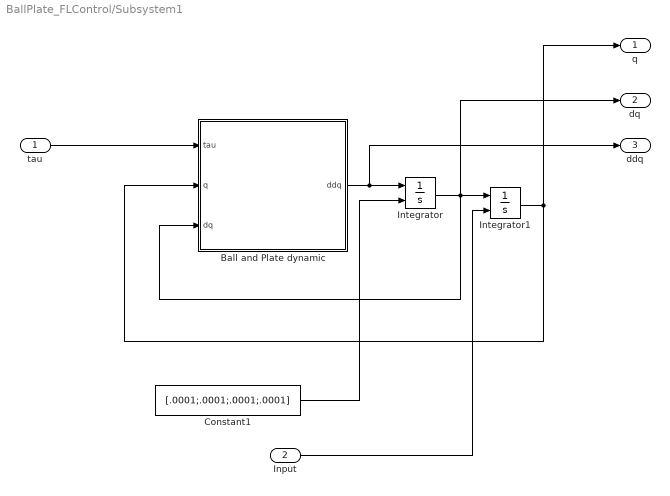
== system BallPlate_FLControl/Subsystem1 ==
  tau : Inport
  Input : Inport  Port=2
  Ball and Plate dynamic : MATLAB Function  TreatAsAtomicUnit=on
  Constant1 : Constant  Value=[.0001;.0001;.0001;.0001]
  Integrator : Integrator  InitialConditionSource=external  InitialCondition=[0;0;0;0]
  Integrator1 : Integrator  InitialConditionSource=external  InitialCondition=[0; 0; 0; 0]
  q : Outport
  dq : Outport  Port=2
  ddq : Outport  Port=3
  wires:
  tau/1 -> Ball and Plate dynamic/1(tau)
  Integrator1/1 -> q/1, Ball and Plate dynamic/2(q)
  Integrator/1 -> dq/1, Integrator1/1, Ball and Plate dynamic/3(dq)
  Ball and Plate dynamic/1(ddq) -> ddq/1, Integrator/1
  Constant1/1 -> Integrator/2
  Input/1 -> Integrator1/2

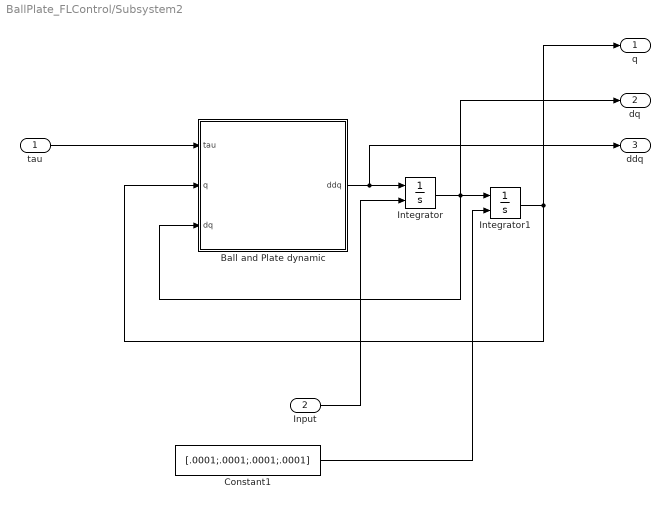
== system BallPlate_FLControl/Subsystem2 ==
  tau : Inport
  Input : Inport  Port=2
  Ball and Plate dynamic : MATLAB Function  TreatAsAtomicUnit=on
  Constant1 : Constant  Value=[.0001;.0001;.0001;.0001]
  Integrator : Integrator  InitialConditionSource=external  InitialCondition=[0;0;0;0]
  Integrator1 : Integrator  InitialConditionSource=external  InitialCondition=[0; 0; 0; 0]
  q : Outport
  dq : Outport  Port=2
  ddq : Outport  Port=3
  wires:
  Constant1/1 -> Integrator1/2
  Input/1 -> Integrator/2
  Ball and Plate dynamic/1(ddq) -> Integrator/1, ddq/1
  Integrator/1 -> Ball and Plate dynamic/3(dq), Integrator1/1, dq/1
  Integrator1/1 -> Ball and Plate dynamic/2(q), q/1
  tau/1 -> Ball and Plate dynamic/1(tau)

== system BallPlate_FLControl/Subsystem3 ==
  In1 : Inport
  In2 : Inport  Port=2
  Gain5 : Gain  Gain=400
  Gain6 : Gain  Gain=1000
  Sum : Sum  Inputs=|++
  Out1 : Outport
  wires:
  Sum/1 -> Out1/1
  Gain6/1 -> Sum/2
  Gain5/1 -> Sum/1
  In2/1 -> Gain6/1
  In1/1 -> Gain5/1

== system BallPlate_FLControl/Subsystem4 ==
  In1 : Inport
  In2 : Inport  Port=2
  Gain5 : Gain  Gain=400
  Gain6 : Gain  Gain=1000
  Sum : Sum  Inputs=|++
  Out1 : Outport
  wires:
  In1/1 -> Gain5/1
  In2/1 -> Gain6/1
  Gain5/1 -> Sum/1
  Gain6/1 -> Sum/2
  Sum/1 -> Out1/1

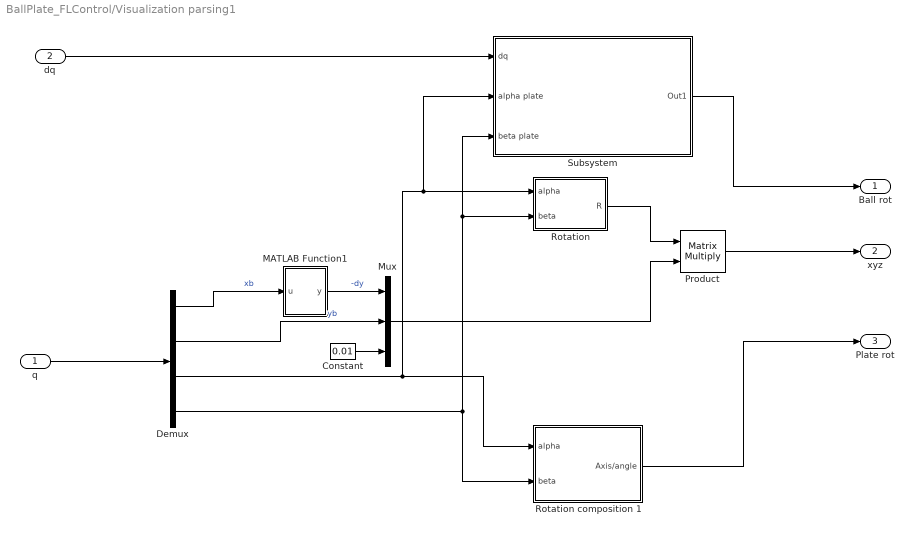
== system BallPlate_FLControl/Visualization parsing1 ==
  q : Inport
  dq : Inport  Port=2
  Constant : Constant  Value=0.01
  Demux : Demux
  MATLAB Function1 : MATLAB Function  TreatAsAtomicUnit=on
  Mux : Mux  Inputs=3
  Product : Product  Multiplication=Matrix(*)
  Rotation : MATLAB Function  TreatAsAtomicUnit=on
  Rotation composition 1 : Subsystem
  Subsystem : Subsystem
  Ball rot : Outport
  xyz : Outport  Port=2
  Plate rot : Outport  Port=3
  wires:
  Demux/2 -> Mux/2  "yb"
  Demux/4 -> Subsystem/3(beta plate), Rotation/2(beta), Rotation composition 1/2(beta)
  Demux/1 -> MATLAB Function1/1(u)  "xb"
  q/1 -> Demux/1
  Demux/3 -> Rotation composition 1/1(alpha), Rotation/1(alpha), Subsystem/2(alpha plate)
  Rotation composition 1/1(Axis/angle) -> Plate rot/1
  Constant/1 -> Mux/3
  Mux/1 -> Product/2
  Rotation/1(R) -> Product/1
  Product/1 -> xyz/1
  dq/1 -> Subsystem/1(dq)
  Subsystem/1(Out1) -> Ball rot/1
  MATLAB Function1/1(y) -> Mux/1  "-dy"

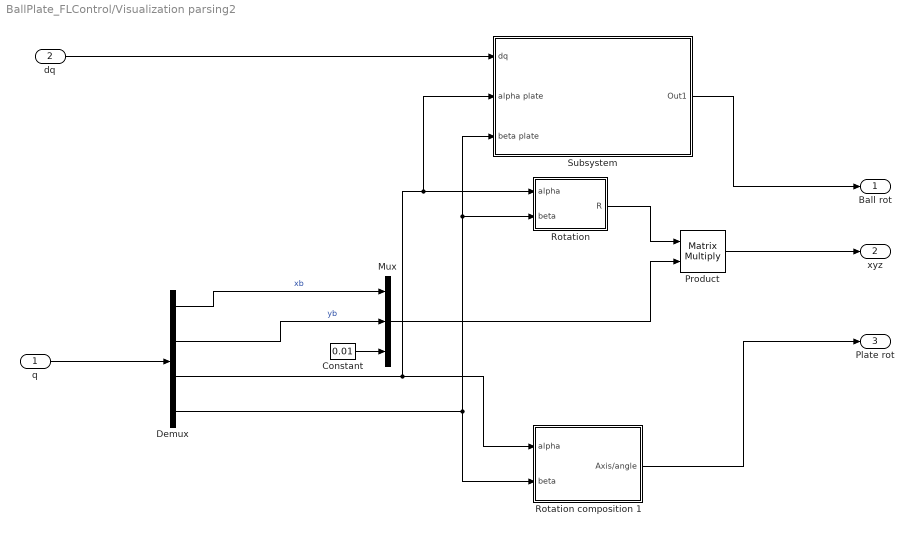
== system BallPlate_FLControl/Visualization parsing2 ==
  q : Inport
  dq : Inport  Port=2
  Constant : Constant  Value=0.01
  Demux : Demux
  Mux : Mux  Inputs=3
  Product : Product  Multiplication=Matrix(*)
  Rotation : MATLAB Function  TreatAsAtomicUnit=on
  Rotation composition 1 : Subsystem
  Subsystem : Subsystem
  Ball rot : Outport
  xyz : Outport  Port=2
  Plate rot : Outport  Port=3
  wires:
  Demux/2 -> Mux/2  "yb"
  Demux/4 -> Subsystem/3(beta plate), Rotation/2(beta), Rotation composition 1/2(beta)
  Demux/1 -> Mux/1  "xb"
  q/1 -> Demux/1
  Demux/3 -> Rotation composition 1/1(alpha), Rotation/1(alpha), Subsystem/2(alpha plate)
  Rotation composition 1/1(Axis/angle) -> Plate rot/1
  Constant/1 -> Mux/3
  Mux/1 -> Product/2
  Rotation/1(R) -> Product/1
  Product/1 -> xyz/1
  dq/1 -> Subsystem/1(dq)
  Subsystem/1(Out1) -> Ball rot/1

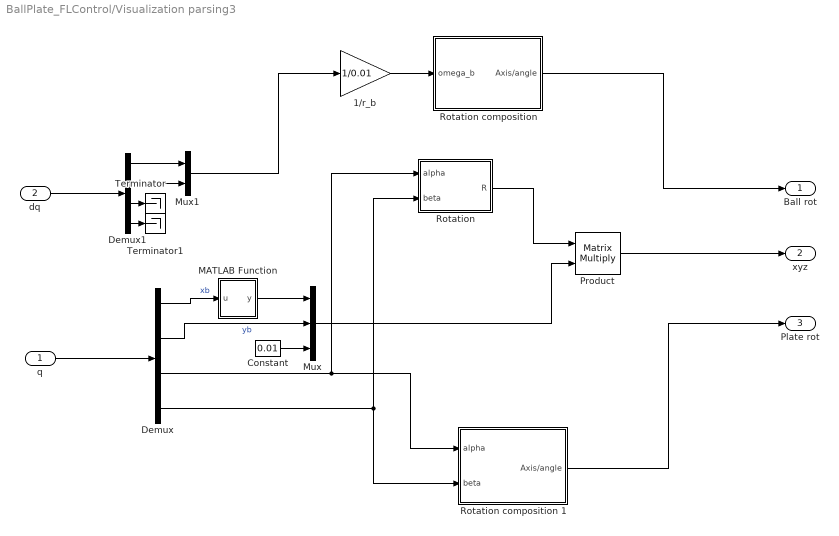
== system BallPlate_FLControl/Visualization parsing3 ==
  q : Inport
  dq : Inport  Port=2
  1/r_b : Gain  Gain=1/0.01
  Constant : Constant  Value=0.01
  Demux : Demux
  Demux1 : Demux
  MATLAB Function : MATLAB Function  TreatAsAtomicUnit=on
  Mux : Mux  Inputs=3
  Mux1 : Mux  Inputs=2
  Product : Product  Multiplication=Matrix(*)
  Rotation : MATLAB Function  TreatAsAtomicUnit=on
  Rotation composition : Subsystem
  Rotation composition 1 : Subsystem
  Terminator : Terminator
  Terminator1 : Terminator
  Ball rot : Outport
  xyz : Outport  Port=2
  Plate rot : Outport  Port=3
  wires:
  Demux/2 -> Mux/2  "yb"
  1/r_b/1 -> Rotation composition/1(omega_b)
  Demux/3 -> Rotation/1(alpha), Rotation composition 1/1(alpha)
  dq/1 -> Demux1/1
  Mux1/1 -> 1/r_b/1
  Demux/1 -> MATLAB Function/1(u)  "xb"
  q/1 -> Demux/1
  Demux1/1 -> Mux1/1
  Demux1/4 -> Terminator1/1
  Rotation composition/1(Axis/angle) -> Ball rot/1
  Demux1/3 -> Terminator/1
  Demux/4 -> Rotation composition 1/2(beta), Rotation/2(beta)
  Rotation composition 1/1(Axis/angle) -> Plate rot/1
  Demux1/2 -> Mux1/2
  Constant/1 -> Mux/3
  Mux/1 -> Product/2
  Rotation/1(R) -> Product/1
  MATLAB Function/1(y) -> Mux/1
  Product/1 -> xyz/1

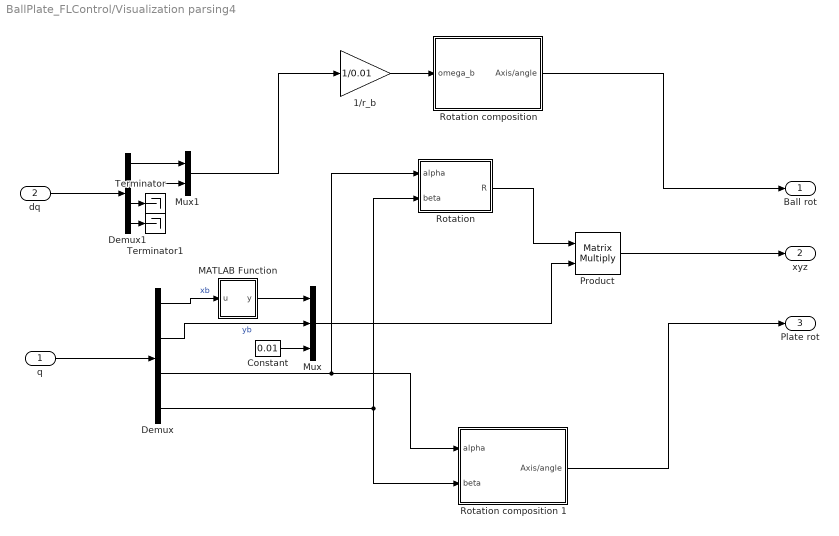
== system BallPlate_FLControl/Visualization parsing4 ==
  q : Inport
  dq : Inport  Port=2
  1/r_b : Gain  Gain=1/0.01
  Constant : Constant  Value=0.01
  Demux : Demux
  Demux1 : Demux
  MATLAB Function : MATLAB Function  TreatAsAtomicUnit=on
  Mux : Mux  Inputs=3
  Mux1 : Mux  Inputs=2
  Product : Product  Multiplication=Matrix(*)
  Rotation : MATLAB Function  TreatAsAtomicUnit=on
  Rotation composition : Subsystem
  Rotation composition 1 : Subsystem
  Terminator : Terminator
  Terminator1 : Terminator
  Ball rot : Outport
  xyz : Outport  Port=2
  Plate rot : Outport  Port=3
  wires:
  Product/1 -> xyz/1
  MATLAB Function/1(y) -> Mux/1
  Rotation/1(R) -> Product/1
  Mux/1 -> Product/2
  Constant/1 -> Mux/3
  Demux1/2 -> Mux1/2
  Rotation composition 1/1(Axis/angle) -> Plate rot/1
  Demux/4 -> Rotation/2(beta), Rotation composition 1/2(beta)
  Demux1/3 -> Terminator/1
  Rotation composition/1(Axis/angle) -> Ball rot/1
  Demux1/4 -> Terminator1/1
  Demux1/1 -> Mux1/1
  q/1 -> Demux/1
  Demux/1 -> MATLAB Function/1(u)  "xb"
  Mux1/1 -> 1/r_b/1
  dq/1 -> Demux1/1
  Demux/3 -> Rotation composition 1/1(alpha), Rotation/1(alpha)
  1/r_b/1 -> Rotation composition/1(omega_b)
  Demux/2 -> Mux/2  "yb"

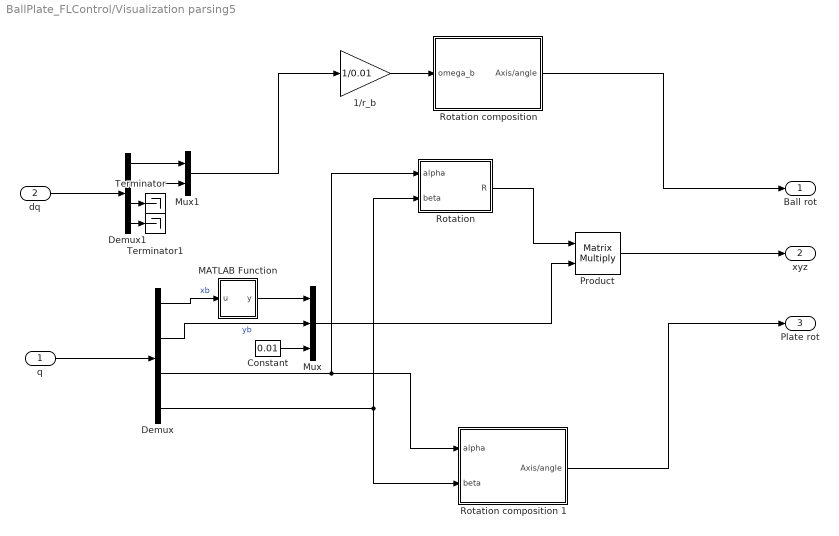
== system BallPlate_FLControl/Visualization parsing5 ==
  q : Inport
  dq : Inport  Port=2
  1/r_b : Gain  Gain=1/0.01
  Constant : Constant  Value=0.01
  Demux : Demux
  Demux1 : Demux
  MATLAB Function : MATLAB Function  TreatAsAtomicUnit=on
  Mux : Mux  Inputs=3
  Mux1 : Mux  Inputs=2
  Product : Product  Multiplication=Matrix(*)
  Rotation : MATLAB Function  TreatAsAtomicUnit=on
  Rotation composition : Subsystem
  Rotation composition 1 : Subsystem
  Terminator : Terminator
  Terminator1 : Terminator
  Ball rot : Outport
  xyz : Outport  Port=2
  Plate rot : Outport  Port=3
  wires:
  Demux/2 -> Mux/2  "yb"
  1/r_b/1 -> Rotation composition/1(omega_b)
  Demux/3 -> Rotation/1(alpha), Rotation composition 1/1(alpha)
  dq/1 -> Demux1/1
  Mux1/1 -> 1/r_b/1
  Demux/1 -> MATLAB Function/1(u)  "xb"
  q/1 -> Demux/1
  Demux1/1 -> Mux1/1
  Demux1/4 -> Terminator1/1
  Rotation composition/1(Axis/angle) -> Ball rot/1
  Demux1/3 -> Terminator/1
  Demux/4 -> Rotation composition 1/2(beta), Rotation/2(beta)
  Rotation composition 1/1(Axis/angle) -> Plate rot/1
  Demux1/2 -> Mux1/2
  Constant/1 -> Mux/3
  Mux/1 -> Product/2
  Rotation/1(R) -> Product/1
  MATLAB Function/1(y) -> Mux/1
  Product/1 -> xyz/1

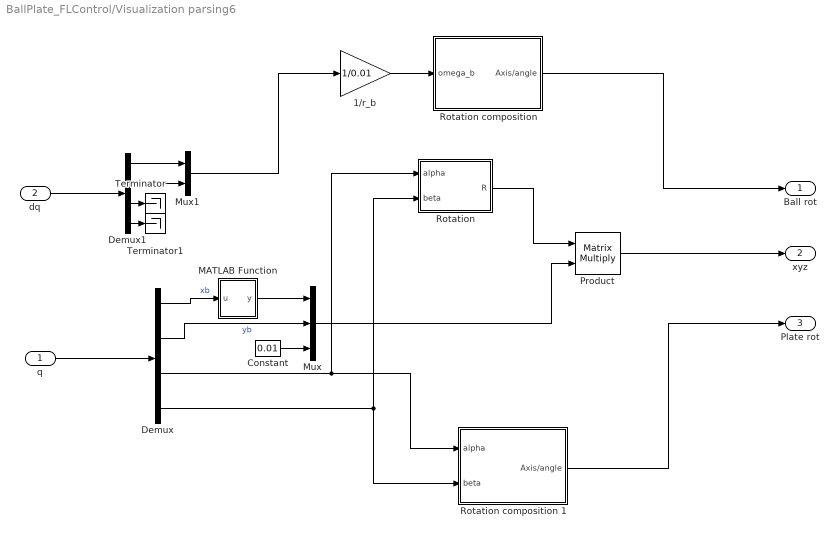
== system BallPlate_FLControl/Visualization parsing6 ==
  q : Inport
  dq : Inport  Port=2
  1/r_b : Gain  Gain=1/0.01
  Constant : Constant  Value=0.01
  Demux : Demux
  Demux1 : Demux
  MATLAB Function : MATLAB Function  TreatAsAtomicUnit=on
  Mux : Mux  Inputs=3
  Mux1 : Mux  Inputs=2
  Product : Product  Multiplication=Matrix(*)
  Rotation : MATLAB Function  TreatAsAtomicUnit=on
  Rotation composition : Subsystem
  Rotation composition 1 : Subsystem
  Terminator : Terminator
  Terminator1 : Terminator
  Ball rot : Outport
  xyz : Outport  Port=2
  Plate rot : Outport  Port=3
  wires:
  Demux/2 -> Mux/2  "yb"
  1/r_b/1 -> Rotation composition/1(omega_b)
  Demux/3 -> Rotation/1(alpha), Rotation composition 1/1(alpha)
  dq/1 -> Demux1/1
  Mux1/1 -> 1/r_b/1
  Demux/1 -> MATLAB Function/1(u)  "xb"
  q/1 -> Demux/1
  Demux1/1 -> Mux1/1
  Demux1/4 -> Terminator1/1
  Rotation composition/1(Axis/angle) -> Ball rot/1
  Demux1/3 -> Terminator/1
  Demux/4 -> Rotation composition 1/2(beta), Rotation/2(beta)
  Rotation composition 1/1(Axis/angle) -> Plate rot/1
  Demux1/2 -> Mux1/2
  Constant/1 -> Mux/3
  Mux/1 -> Product/2
  Rotation/1(R) -> Product/1
  MATLAB Function/1(y) -> Mux/1
  Product/1 -> xyz/1

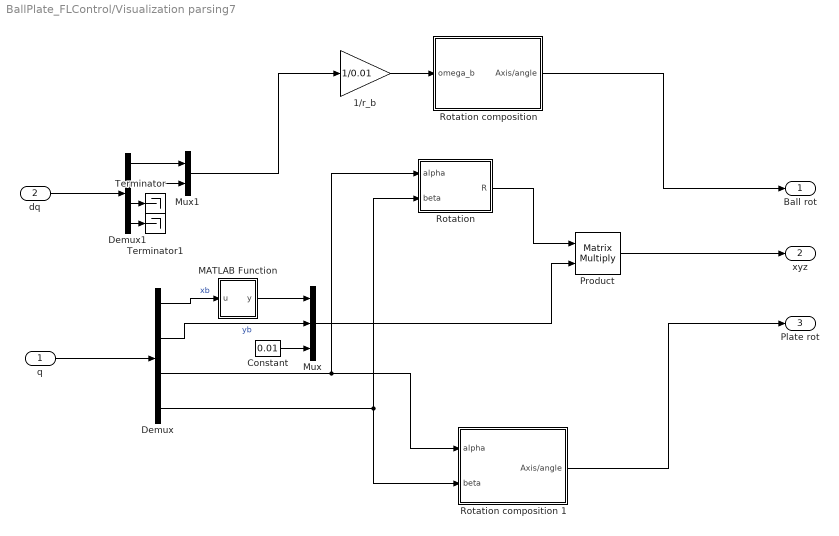
== system BallPlate_FLControl/Visualization parsing7 ==
  q : Inport
  dq : Inport  Port=2
  1/r_b : Gain  Gain=1/0.01
  Constant : Constant  Value=0.01
  Demux : Demux
  Demux1 : Demux
  MATLAB Function : MATLAB Function  TreatAsAtomicUnit=on
  Mux : Mux  Inputs=3
  Mux1 : Mux  Inputs=2
  Product : Product  Multiplication=Matrix(*)
  Rotation : MATLAB Function  TreatAsAtomicUnit=on
  Rotation composition : Subsystem
  Rotation composition 1 : Subsystem
  Terminator : Terminator
  Terminator1 : Terminator
  Ball rot : Outport
  xyz : Outport  Port=2
  Plate rot : Outport  Port=3
  wires:
  Product/1 -> xyz/1
  MATLAB Function/1(y) -> Mux/1
  Rotation/1(R) -> Product/1
  Mux/1 -> Product/2
  Constant/1 -> Mux/3
  Demux1/2 -> Mux1/2
  Rotation composition 1/1(Axis/angle) -> Plate rot/1
  Demux/4 -> Rotation/2(beta), Rotation composition 1/2(beta)
  Demux1/3 -> Terminator/1
  Rotation composition/1(Axis/angle) -> Ball rot/1
  Demux1/4 -> Terminator1/1
  Demux1/1 -> Mux1/1
  q/1 -> Demux/1
  Demux/1 -> MATLAB Function/1(u)  "xb"
  Mux1/1 -> 1/r_b/1
  dq/1 -> Demux1/1
  Demux/3 -> Rotation composition 1/1(alpha), Rotation/1(alpha)
  1/r_b/1 -> Rotation composition/1(omega_b)
  Demux/2 -> Mux/2  "yb"

== system BallPlate_FLControl/Feedback linearized /Feedback Linearization ==
  nu : Inport
  q : Inport  Port=2
  dq : Inport  Port=3
  Einv_matrix : MATLAB Function  TreatAsAtomicUnit=on
  Gamma_matrix : MATLAB Function  TreatAsAtomicUnit=on
  Matrix Multiply : Product  Multiplication=Matrix(*)
  Matrix Multiply1 : Product  Multiplication=Matrix(*)
  Sum : Sum  Inputs=+-
  u : Outport
  wires:
  q/1 -> Gamma_matrix/1(q), Einv_matrix/1(q)
  dq/1 -> Gamma_matrix/2(dq), Einv_matrix/2(dq)
  Einv_matrix/1(Einv) -> Matrix Multiply1/1, Matrix Multiply/1
  nu/1 -> Matrix Multiply/2
  Gamma_matrix/1(Gamma) -> Matrix Multiply1/2
  Matrix Multiply/1 -> Sum/1
  Matrix Multiply1/1 -> Sum/2
  Sum/1 -> u/1

== system BallPlate_FLControl/Feedback linearized /Subsystem ==
  tau : Inport
  Ball and Plate dynamic : MATLAB Function  TreatAsAtomicUnit=on
  Constant : Constant  Value=[0.0001;0.0001;.0001;.0001]
  Constant1 : Constant  Value=[.0001;.0001;.0001;.0001]
  Integrator : Integrator  InitialConditionSource=external  InitialCondition=[0;0;0;0]
  Integrator1 : Integrator  InitialConditionSource=external  InitialCondition=[0; 0; 0; 0]
  q : Outport
  dq : Outport  Port=2
  wires:
  tau/1 -> Ball and Plate dynamic/1(tau)
  Integrator1/1 -> q/1, Ball and Plate dynamic/2(q)
  Integrator/1 -> dq/1, Integrator1/1, Ball and Plate dynamic/3(dq)
  Ball and Plate dynamic/1(ddq) -> Integrator/1
  Constant/1 -> Integrator/2
  Constant1/1 -> Integrator1/2

== system BallPlate_FLControl/Feedback linearized 1/Feedback Linearization ==
  nu : Inport
  q : Inport  Port=2
  dq : Inport  Port=3
  Einv_matrix : MATLAB Function  TreatAsAtomicUnit=on
  Gamma_matrix : MATLAB Function  TreatAsAtomicUnit=on
  Matrix Multiply : Product  Multiplication=Matrix(*)
  Matrix Multiply1 : Product  Multiplication=Matrix(*)
  Sum : Sum  Inputs=+-
  u : Outport
  wires:
  Sum/1 -> u/1
  Matrix Multiply1/1 -> Sum/2
  Matrix Multiply/1 -> Sum/1
  Gamma_matrix/1(Gamma) -> Matrix Multiply1/2
  nu/1 -> Matrix Multiply/2
  Einv_matrix/1(Einv) -> Matrix Multiply/1, Matrix Multiply1/1
  dq/1 -> Einv_matrix/2(dq), Gamma_matrix/2(dq)
  q/1 -> Einv_matrix/1(q), Gamma_matrix/1(q)

== system BallPlate_FLControl/Feedback linearized 1/Subsystem ==
  tau : Inport
  Ball and Plate dynamic : MATLAB Function  TreatAsAtomicUnit=on
  Constant : Constant  Value=[0.0001;0.0001;.0001;.0001]
  Constant1 : Constant  Value=[.0001;.0001;.0001;.0001]
  Integrator : Integrator  InitialConditionSource=external  InitialCondition=[0;0;0;0]
  Integrator1 : Integrator  InitialConditionSource=external  InitialCondition=[0; 0; 0; 0]
  q : Outport
  dq : Outport  Port=2
  wires:
  Constant1/1 -> Integrator1/2
  Constant/1 -> Integrator/2
  Ball and Plate dynamic/1(ddq) -> Integrator/1
  Integrator/1 -> Ball and Plate dynamic/3(dq), Integrator1/1, dq/1
  Integrator1/1 -> Ball and Plate dynamic/2(q), q/1
  tau/1 -> Ball and Plate dynamic/1(tau)

== system BallPlate_FLControl/Feedback linearized 2/Feedback Linearization ==
  nu : Inport
  q : Inport  Port=2
  dq : Inport  Port=3
  Einv_matrix : MATLAB Function  TreatAsAtomicUnit=on
  Gamma_matrix : MATLAB Function  TreatAsAtomicUnit=on
  Matrix Multiply : Product  Multiplication=Matrix(*)
  Matrix Multiply1 : Product  Multiplication=Matrix(*)
  Sum : Sum  Inputs=+-
  u : Outport
  wires:
  q/1 -> Gamma_matrix/1(q), Einv_matrix/1(q)
  dq/1 -> Gamma_matrix/2(dq), Einv_matrix/2(dq)
  Einv_matrix/1(Einv) -> Matrix Multiply1/1, Matrix Multiply/1
  nu/1 -> Matrix Multiply/2
  Gamma_matrix/1(Gamma) -> Matrix Multiply1/2
  Matrix Multiply/1 -> Sum/1
  Matrix Multiply1/1 -> Sum/2
  Sum/1 -> u/1

== system BallPlate_FLControl/Feedback linearized 2/Subsystem ==
  tau : Inport
  "p0 " : Inport  Port=2
  Ball and Plate dynamic : MATLAB Function  TreatAsAtomicUnit=on
  Constant : Constant  Value=[0.0001;0.0001;.0001;.0001]
  Integrator : Integrator  InitialConditionSource=external  InitialCondition=[0;0;0;0]
  Integrator1 : Integrator  InitialConditionSource=external  InitialCondition=[0; 0; 0; 0]
  q : Outport
  dq : Outport  Port=2
  wires:
  tau/1 -> Ball and Plate dynamic/1(tau)
  Integrator1/1 -> q/1, Ball and Plate dynamic/2(q)
  Integrator/1 -> dq/1, Integrator1/1, Ball and Plate dynamic/3(dq)
  Ball and Plate dynamic/1(ddq) -> Integrator/1
  Constant/1 -> Integrator/2
  "p0 "/1 -> Integrator1/2

== system BallPlate_FLControl/Feedback linearized 3/Feedback Linearization ==
  nu : Inport
  q : Inport  Port=2
  dq : Inport  Port=3
  Einv_matrix : MATLAB Function  TreatAsAtomicUnit=on
  Gamma_matrix : MATLAB Function  TreatAsAtomicUnit=on
  Matrix Multiply : Product  Multiplication=Matrix(*)
  Matrix Multiply1 : Product  Multiplication=Matrix(*)
  Sum : Sum  Inputs=+-
  u : Outport
  wires:
  q/1 -> Gamma_matrix/1(q), Einv_matrix/1(q)
  dq/1 -> Gamma_matrix/2(dq), Einv_matrix/2(dq)
  Einv_matrix/1(Einv) -> Matrix Multiply1/1, Matrix Multiply/1
  nu/1 -> Matrix Multiply/2
  Gamma_matrix/1(Gamma) -> Matrix Multiply1/2
  Matrix Multiply/1 -> Sum/1
  Matrix Multiply1/1 -> Sum/2
  Sum/1 -> u/1
